simulink model "LaserModel"  (R2020a)
settings: Solver=VariableStepAuto  StartTime=0.0  StopTime=10.0  RelTol=1e-3
settings Model: Creator=MSI  LastModifiedBy=MSI

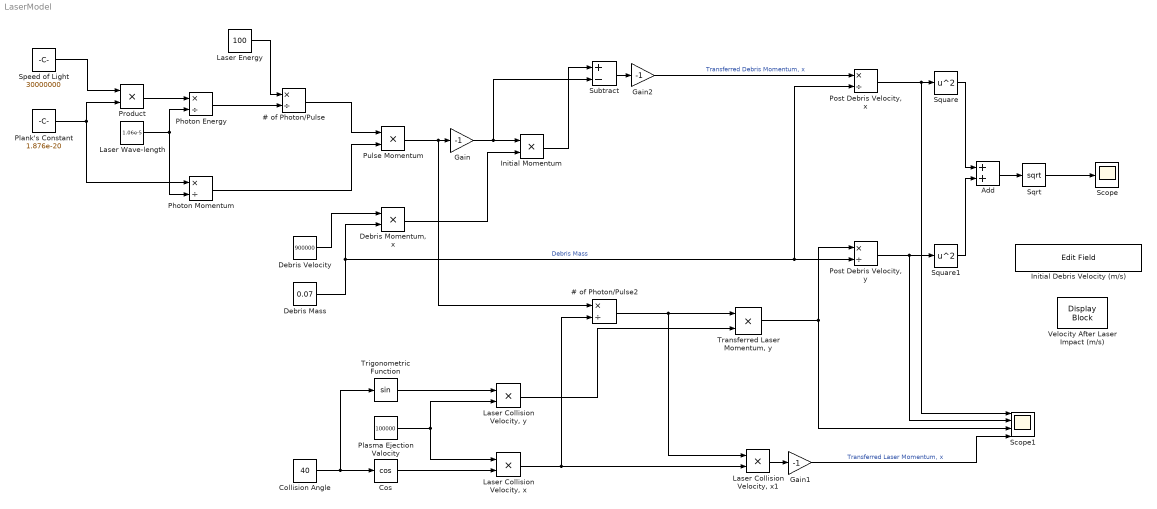
== system LaserModel ==
  " Transferred Laser Momentum, y" : Product
  # of Photon/Pulse : Product  Inputs=*/
  # of Photon/Pulse2 : Product  Inputs=*/
  Add : Sum
  Collision Angle : Constant  Value=40  OutDataTypeStr=Inherit: Inherit via back propagation
  Cos : Trigonometry  Operator=cos
  Debris Mass : Constant  Value=0.07  OutDataTypeStr=Inherit: Inherit via back propagation
  "Debris Momentum, x" : Product
  Debris Velocity : Constant  Value=900000  OutDataTypeStr=Inherit: Inherit via back propagation
  Gain : Gain  Gain=-1
  Gain1 : Gain  Gain=-1
  Gain2 : Gain  Gain=-1
  Initial Debris Velocity (m/s) : EditField  LabelPosition=Hide  ShowInitialText=on  Alignment=Center
  Initial Momentum : Product
  "Laser Collision Velocity, x" : Product
  "Laser Collision Velocity, x1" : Product
  "Laser Collision Velocity, y" : Product
  Laser Energy : Constant  Value=100  OutDataTypeStr=Inherit: Inherit via back propagation
  Laser Wave-length : Constant  Value=1.06e-5  OutDataTypeStr=Inherit: Inherit via back propagation
  Photon Energy : Product  Inputs=*/
  Photon Momentum : Product  Inputs=*/
  Plank's Constant : Constant  Value=1.876e-20  OutDataTypeStr=Inherit: Inherit via back propagation
  Plasma Ejection Valocity : Constant  Value=100000  OutDataTypeStr=Inherit: Inherit via back propagation
  "Post Debris Velocity, x" : Product  Inputs=*/
  "Post Debris Velocity, y" : Product  Inputs=*/
  Product : Product
  Pulse Momentum : Product
  Scope : Scope
  Scope1 : Scope  NumInputPorts=4
  Speed of Light : Constant  Value=30000000  OutDataTypeStr=Inherit: Inherit via back propagation
  Sqrt : Sqrt  SaturateOnIntegerOverflow=on
  Square : Math  Operator=square  SaturateOnIntegerOverflow=on
  Square1 : Math  Operator=square  SaturateOnIntegerOverflow=on
  Subtract : Sum  Inputs=+-
  Trigonometric Function : Trigonometry
  Velocity After Laser Impact (m/s) : DisplayBlock  LabelPosition=Hide  Format=short  Transparency=1
  wires:
  Speed of Light/1 -> Product/1
  Plank's Constant/1 -> Photon Momentum/1, Product/2
  Product/1 -> Photon Energy/1
  Laser Wave-length/1 -> Photon Momentum/2, Photon Energy/2
  Laser Energy/1 -> # of Photon/Pulse/1
  Photon Energy/1 -> # of Photon/Pulse/2
  # of Photon/Pulse/1 -> Pulse Momentum/1
  Photon Momentum/1 -> Pulse Momentum/2
  Pulse Momentum/1 -> # of Photon/Pulse2/1, Gain/1
  Gain/1 -> Subtract/2, Initial Momentum/1
  Debris Mass/1 -> "Post Debris Velocity, x"/2, "Post Debris Velocity, y"/2, "Debris Momentum, x"/2  "Debris Mass"
  Debris Velocity/1 -> "Debris Momentum, x"/1
  "Debris Momentum, x"/1 -> Initial Momentum/2
  Initial Momentum/1 -> Subtract/1
  Subtract/1 -> Gain2/1
  Gain2/1 -> "Post Debris Velocity, x"/1  "Transferred Debris Momentum, x"
  Collision Angle/1 -> Cos/1, Trigonometric Function/1
  Cos/1 -> "Laser Collision Velocity, x"/2
  Plasma Ejection Valocity/1 -> "Laser Collision Velocity, x"/1, "Laser Collision Velocity, y"/2
  Trigonometric Function/1 -> "Laser Collision Velocity, y"/1
  "Laser Collision Velocity, x"/1 -> # of Photon/Pulse2/2, "Laser Collision Velocity, x1"/2
  # of Photon/Pulse2/1 -> "Laser Collision Velocity, x1"/1, " Transferred Laser Momentum, y"/1
  "Laser Collision Velocity, y"/1 -> " Transferred Laser Momentum, y"/2
  "Laser Collision Velocity, x1"/1 -> Gain1/1
  "Post Debris Velocity, x"/1 -> Scope1/1, Square/1
  " Transferred Laser Momentum, y"/1 -> Scope1/3, "Post Debris Velocity, y"/1
  "Post Debris Velocity, y"/1 -> Scope1/2, Square1/1
  Square/1 -> Add/1
  Square1/1 -> Add/2
  Add/1 -> Sqrt/1
  Sqrt/1 -> Scope/1
  Gain1/1 -> Scope1/4  "Transferred Laser Momentum, x"
